simulink model "P2_19"  (R2015b)
settings: Solver=VariableStepAuto  StartTime=0.0  StopTime=1  MaxStep=.01  RelTol=1e-3
settings Model: Creator=sam  LastModifiedBy=sam

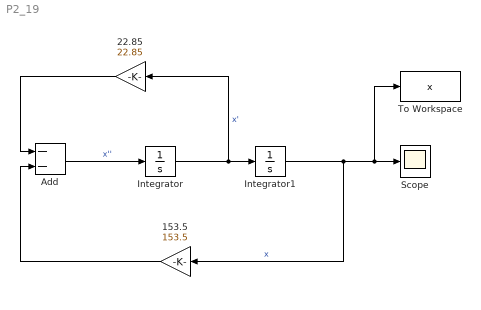
== system P2_19 ==
  153.5 : Gain  Gain=153.5
  22.85 : Gain  Gain=22.85
  Add : Sum  Inputs=--
  Integrator : Integrator
  Integrator1 : Integrator  InitialCondition=.05236
  Scope : Scope
  To Workspace : ToWorkspace  VariableName=x  SaveFormat=Timeseries  SampleTime=-1
  wires:
  Add/1 -> Integrator/1  "x''"
  Integrator/1 -> 22.85/1, Integrator1/1  "x'"
  Integrator1/1 -> 153.5/1, To Workspace/1, Scope/1  "x"
  22.85/1 -> Add/1
  153.5/1 -> Add/2
